simulink model "feedback"  (R2017a)
settings: Solver=VariableStepAuto  StartTime=0.0  StopTime=10.0  RelTol=1e-3
settings Model: Creator=TUDelft SID  LastModifiedBy=TUDelft SID

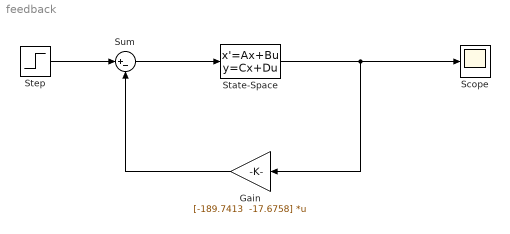
== system feedback ==
  Gain : Gain  Gain="[-189.7413  -17.6758]"  Multiplication=Matrix(K*u)
      mask Display: disp('K*u')
  Scope : Scope
  State-Space : StateSpace  A=|  B=|  C=|  D=[0;0]  X0=0
      A=|
      | [-0.974838327898342, 0.950496207114418;
      | -4.27636880764243, -1.31742910049042]
      B=|
      | [-0.00204980648923711;
      | -0.313898672488684]
      C=|
      | [57.2957795130823, 0;
      | 0, 57.2957795130823]
  Step : Step  SampleTime=0
  Sum : Sum  Inputs=|+-
  wires:
  State-Space/1 -> Gain/1, Scope/1
  Gain/1 -> Sum/2
  Sum/1 -> State-Space/1
  Step/1 -> Sum/1
